simulink model "wetmodel"  (R2020b)
settings: Solver=ode45  StartTime=0.0  StopTime=inf  RelTol=1e-3  EnableMultiTasking=on
values from neighbouring files (symbols this model uses):
  controller = evalin('base','controller')    [setting_editor.m]
  s = evalin('base','s')    [GUI_MT44001.m]
undefined symbols (not defined in the file or in its folder): TS_boat
libraries: dsparch4 x6, slctrlblks x3, simulink x2, robotlib x1, dspsigops x1, aerolibutil x1
settings Model: Tag=MP_system  EnablePacing=on  Creator=Andries  LastModifiedBy=jurre
settings DataIOCC: LimitDataPoints=on  SaveFormat=Array  SignalLoggingSaveFormat=ModelDataLogs  ReturnWorkspaceOutputs=off
settings OptimizationCC: ExpressionDepthLimit=2147483647  LifeSpan=inf
settings DebuggingCC: UnderspecifiedInitializationDetection=Classic  MergeDetectMultiDrivingBlocksExec=none  SolverPrmCheckMsg=warning  FcnCallInpInsideContextMsg=warning  StateNameClashWarn=warning  SFUnexpectedBacktrackingDiag=warning  SFNoUnconditionalDefaultTransitionDiag=warning  SFExecutionAtInitializationDiag=none  ArithmeticOperatorsInVariantConditions=warning
settings HardwareCC: ProdBitPerPointer=32  ProdBitPerSizeT=32  ProdBitPerPtrDiffT=32  ProdLargestAtomicFloat=None  ProdIntDivRoundTo=Undefined  ProdEndianess=Unspecified  ProdWordSize=32  ProdHWDeviceType=32-bit Generic
settings ModelReferenceCC: PropagateSignalLabelsOutOfModel=off
settings SFSimCC: SimUseLocalCustomCode=off  CustomCodeUndefinedFunction=UseInterfaceOnly
settings RTWCC: RTWUseLocalCustomCode=off
settings CodeAppCC: StateflowObjectComments=on
settings GRTTargetCC: TargetLangStandard=C89/C90 (ANSI)  CombineOutputUpdateFcns=off  GRTInterface=on
settings ConfigComp: CovMetricSettings=dw  CovSaveCumulativeToWorkspaceVar=on  CovSaveSingleToWorkspaceVar=on  CovExternalEMLEnable=off
settings SimscapeCC: SimscapeNormalizeSystem=off

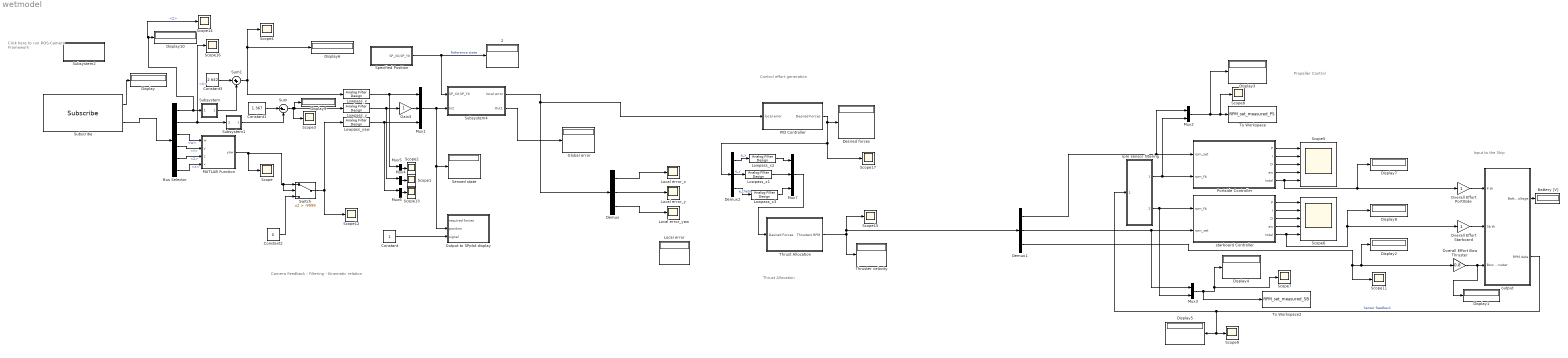
== system wetmodel ==
  note: Camera Feedback - Filtering - Kinematic relation
  note: Control effort generation
  note: Thrust Allocation
  note: Input to the Ship
  note: Propeller Control
  note: Click here to run
      | ROS-Camera Framework
  "  2" : Display
  Battery [V] : Display
  Bus Selector : BusSelector  OutputSignals=Pose.Position.Z,Pose.Position.X,Pose.Orientation.W,Pose.Orientation.Y,Pose.Orientation.Z,Pose.Orientation.X
  Constant : Constant
  Constant1 : Constant  Value=1.367
  Constant2 : Constant  Value=0
  Constant3 : Constant  Value=2.642
  Demux : Demux  Outputs=3
  Demux1 : Demux  Outputs=3
  Demux2 : Demux  Outputs=3
  Desired forces : Display
  Display{,1..10} (11 alike) : Display
  Gain3 : Gain
  Global error : Display
  Local error : Display
  "Local error_x " : Scope
  "Local error_y " : Scope
  "Local error_yaw " : Scope
  Lowpass_x{,1..3} (4 alike) : dsparch4/Analog Filter Design  method=Butterworth  filttype=Lowpass  N=1  Wlo=30  Whi=80  Rp=2  Rs=40
  Lowpass_y : dsparch4/Analog Filter Design  method=Butterworth  filttype=Lowpass  N=1  Wlo=30  Whi=80  Rp=2  Rs=40
  Lowpass_yaw : dsparch4/Analog Filter Design  method=Butterworth  filttype=Lowpass  N=8  Wlo=30  Whi=80  Rp=2  Rs=40
  MATLAB Function : MATLAB Function  TreatAsAtomicUnit=on
  Mux1 : Mux  Inputs=3
  Mux{2..6} (5 alike) : Mux  Inputs=2
  Mux7 : Mux  Inputs=3
  Output to SPplot display : Subsystem
      mask Display:
      | image(imread('spplot.JPG'))
      | port_label('input', 1, 'Req. Forces')
      | port_label('input', 2, 'Pos Update')
      | port_label('input', 3, 'signal')
  Overall Effort Bow Thruster : Gain  Gain=0.8
  Overall Effort PortISide : Gain
  Overall Effort Starboard : Gain
  PID Controller : Subsystem
  Portside Controller : Subsystem  mask{P=controller.PP, I=controller.PI, D=controller.PD, P_aw=controller.PPaw}
      mask help: Controller setting for Starboard engine
  Scope{,1..4,7..9,11..17} (15 alike) : Scope
  Scope5 : Scope  NumInputPorts=5
  Scope6 : Scope  NumInputPorts=5
  Sensed state : Display
  Specified Position : Subsystem
  Subscribe : robotlib/Subscribe  topicSource=Select from ROS network  topic=/OptiRAS/RAS_TN_RE/pose  messageType=geometry_msgs/PoseStamped  SampleTime=-1  legacyBusStruct=off  messageQueueLength=1
  Subsystem : Subsystem
  Subsystem1 : Subsystem
  Subsystem2 : Subsystem  InitFcn=|  StopFcn=set_param(gcb,'BackgroundColor','red');
      | %if ros_init==1
      | if ros.internal.Global.isNodeActive == 1
      | set_param(gcb,'BackgroundColor','green');
      | else
      | set_param(gcb,'BackgroundColor','red');
      | end
      settings: ModelCloseFcn=set_param(gcb,'BackgroundColor','red');  CloseFcn=set_param(gcb,'BackgroundColor','red');
  Subsystem4 : Subsystem
  Sum : Sum  Inputs=|+-
  Sum1 : Sum  Inputs=|++
  Switch : Switch  Criteria=u2 > Threshold  Threshold=-9999
  Thrust Allocation : Subsystem
  Thruster velocity : Display
  To Workspace : ToWorkspace  VariableName=RPM_set_measured_PS  SampleTime=-1
  To Workspace2 : ToWorkspace  VariableName=RPM_set_measured_SB  SampleTime=-1
  output : Subsystem
  rpm sensor filtering : Subsystem  mask{n_p=controller.Prpm, n_sb=controller.STrpm}
      mask prompts: n_p "Amount of holes in portside RPM sensor disc"; n_sb "Amount of holes in portside RPM sensor disc"
      mask Display:
      | port_label('output', 1, 'Ps RPM')
      | port_label('output', 2, 'SBs RPM')
  starboard Controller : Subsystem  mask{P=controller.STP, I=controller.STI, D=controller.STD, P_aw=controller.STPaw}
      mask help: Controller setting for Starboard engine
  wires:
  Specified Position/1(SP_X0,SP_Y0) -> Subsystem4/1(SP_X0,SP_Y0), "  2"/1  "Reference state"
  Mux1/1 -> Subsystem4/2(In2), Output to SPplot display/2(position), Sensed state/1
  output/2(RPM data) -> Scope9/1, Display5/1, rpm sensor filtering/1(RPM data)  "Sensor feedback"
  Portside Controller/4(aw) -> Scope5/4
  starboard Controller/3(D) -> Scope6/3
  output/1(Battery voltage) -> Battery [V]/1
  rpm sensor filtering/1(portside rpm) -> Mux2/2, Portside Controller/2(rpm_fb)
  Portside Controller/1(" P") -> Scope5/1
  rpm sensor filtering/2(starboard side rpm) -> starboard Controller/1(rpm_fb), Mux3/2
  Mux2/1 -> To Workspace/1, Scope8/1, Display3/1
  Portside Controller/3(D) -> Scope5/3
  starboard Controller/4(aw) -> Scope6/4
  Mux3/1 -> To Workspace2/1, Display4/1, Scope7/1
  Portside Controller/2(I) -> Scope5/2
  starboard Controller/2(I) -> Scope6/2
  starboard Controller/1(" P") -> Scope6/1
  Demux1/1 -> Mux2/1, Portside Controller/1(rpm_set)
  Portside Controller/5(total) -> Scope5/5, Overall Effort PortISide/1, Display7/1
  Demux1/2 -> starboard Controller/2(rpm_set), Mux3/1
  Demux1/3 -> Overall Effort Bow Thruster/1, Display2/1, Scope11/1
  Overall Effort PortISide/1 -> output/1(P th)
  Overall Effort Starboard/1 -> output/2(Sb th)
  Lowpass_x/1 -> Mux1/1, Mux5/1
  Lowpass_y/1 -> Mux4/1, Gain3/1
  Lowpass_yaw/1 -> Mux1/3, Mux6/1
  Thrust Allocation/1(Thrusters RPM) -> Demux1/1, Scope15/1, Thruster velocity/1
  PID Controller/1(Desired Forces) -> Demux2/1, Scope17/1, Desired forces/1
  Mux6/1 -> Scope13/1
  Mux4/1 -> Scope1/1
  Mux5/1 -> Scope2/1
  starboard Controller/5(total) -> Scope6/5, Overall Effort Starboard/1, Display8/1
  Overall Effort Bow Thruster/1 -> output/3("Bow thruster "), Display1/1
  Subscribe/1 -> Display/1
  Subscribe/2 -> Bus Selector/1
  Constant/1 -> Output to SPplot display/3(signal)
  Bus Selector/3 -> MATLAB Function/1(w)  "<W>"
  Bus Selector/4 -> MATLAB Function/2(y)  "<Y>"
  Bus Selector/5 -> MATLAB Function/3(z)  "<Z>"
  Bus Selector/6 -> MATLAB Function/4(x)  "<X>"
  MATLAB Function/1(yaw) -> Switch/2, Switch/1, Scope/1
  Switch/1 -> Lowpass_yaw/1, Scope12/1
  Constant2/1 -> Switch/3
  Sum/1 -> Scope3/1, Lowpass_y/1, Display9/1
  Constant1/1 -> Sum/1
  Sum1/1 -> Scope4/1, Display6/1, Lowpass_x/1
  Constant3/1 -> Sum1/1
  Bus Selector/1 -> Scope14/1, Display10/1, Subsystem/1(In1)  "<Z>"
  Bus Selector/2 -> Subsystem1/1(In1), Scope16/1  "<X>"
  Subsystem/1(Out1) -> Sum1/2
  Subsystem1/1(Out1) -> Sum/2
  Demux2/2 -> Lowpass_x1/1  "e_y"
  Demux2/3 -> Lowpass_x3/1  "e_theta"
  Lowpass_x3/1 -> Mux7/3
  Lowpass_x1/1 -> Mux7/2
  Lowpass_x2/1 -> Mux7/1
  Demux2/1 -> Lowpass_x2/1  "e_x"
  Mux7/1 -> Thrust Allocation/1(Desired Forces)
  Gain3/1 -> Mux1/2
  Subsystem4/1(local error) -> Demux/1, PID Controller/1(local error)
  Demux/1 -> "Local error_x "/1
  Demux/2 -> "Local error_y "/1
  Demux/3 -> "Local error_yaw "/1
  Subsystem4/2(Out1) -> Global error/1

== system wetmodel/Output to SPplot display ==
  required forces : Inport
  position : Inport  Port=2
  signal : Inport  Port=3
  Constant : Constant  Value=3
  Mux : Mux  Inputs=3
  Switch : Switch  Criteria=u2 > Threshold
  pos_update : S-Function  FunctionName=pos_update  Parameters=TS_wii  SFunctionDeploymentMode=off  EnableBusSupport=off
  wires:
  Mux/1 -> pos_update/1
  position/1 -> Mux/1
  required forces/1 -> Mux/3
  Switch/1 -> Mux/2
  signal/1 -> Switch/2
  Constant/1 -> Switch/1

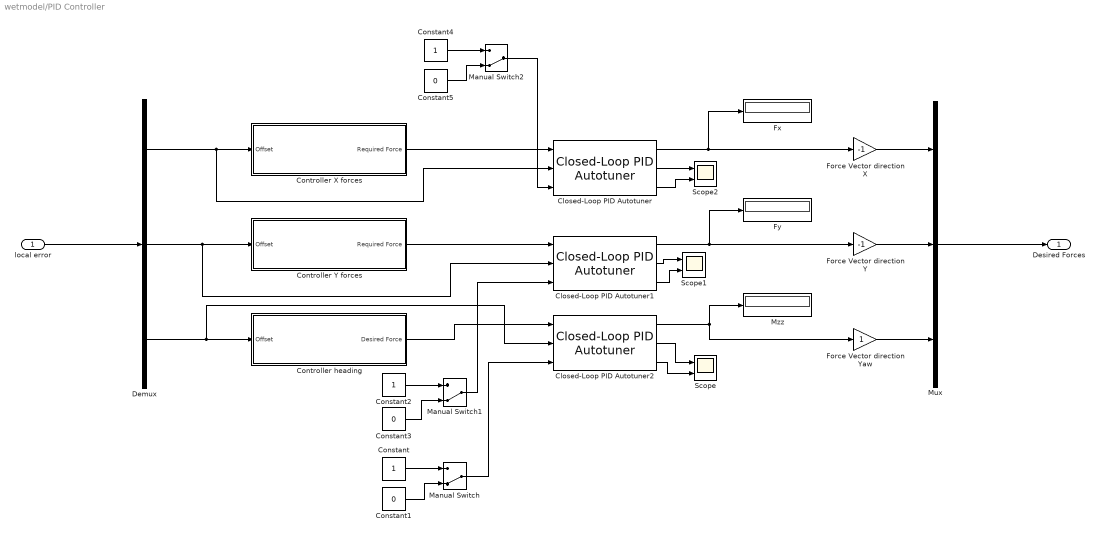
== system wetmodel/PID Controller ==
  local error : Inport
  Closed-Loop PID Autotuner : slctrlblks/Closed-Loop PID Autotuner  PIDType=PID  PIDForm=Parallel  TimeDomain=continuous-time  DiscreteTs=0.1  IntegratorFormula=Forward Euler  FilterFormula=Forward Euler  ContinuousTs=0.02  Bandwidth=1  UseExternalWC=off  TargetPM=60  UseExternalPM=off  UseExternalAchievedPM=off  PlantType=Stable  PlantSign=Positive  AmpSine=1  UseExternalAmpSine=off  UseExternalFRD=off  UseExternalU0=off  UseCompanion=off  NotDeployTuningModule=off  UsePLCCoder=off  OutputMode=control action + perturbation  BlockDataType=double  UseConnectedPID=on  blockpath=[]  tunedP=0  tunedI=0  tunedD=0  tunedN=100  tunedPM=0  EstimationWindowSize=3  UseExternalTuningParams=off  OutputChoice=VariantCandD
      settings: SourceProductBaseCode=SD
  Closed-Loop PID Autotuner1 : slctrlblks/Closed-Loop PID Autotuner  PIDType=PID  PIDForm=Parallel  TimeDomain=continuous-time  DiscreteTs=0.1  IntegratorFormula=Forward Euler  FilterFormula=Forward Euler  ContinuousTs=0.02  Bandwidth=1  UseExternalWC=off  TargetPM=60  UseExternalPM=off  UseExternalAchievedPM=off  PlantType=Stable  PlantSign=Positive  AmpSine=1  UseExternalAmpSine=off  UseExternalFRD=off  UseExternalU0=off  UseCompanion=off  NotDeployTuningModule=off  UsePLCCoder=off  OutputMode=control action + perturbation  BlockDataType=double  UseConnectedPID=on  blockpath=[]  tunedP=0  tunedI=0  tunedD=0  tunedN=100  tunedPM=0  EstimationWindowSize=3  UseExternalTuningParams=off  OutputChoice=VariantCandD
      settings: SourceProductBaseCode=SD
  Closed-Loop PID Autotuner2 : slctrlblks/Closed-Loop PID Autotuner  PIDType=PID  PIDForm=Parallel  TimeDomain=continuous-time  DiscreteTs=0.1  IntegratorFormula=Forward Euler  FilterFormula=Forward Euler  ContinuousTs=0.02  Bandwidth=1  UseExternalWC=off  TargetPM=60  UseExternalPM=off  UseExternalAchievedPM=off  PlantType=Stable  PlantSign=Positive  AmpSine=1  UseExternalAmpSine=off  UseExternalFRD=off  UseExternalU0=off  UseCompanion=off  NotDeployTuningModule=off  UsePLCCoder=off  OutputMode=control action + perturbation  BlockDataType=double  UseConnectedPID=on  blockpath=[]  tunedP=0  tunedI=0  tunedD=0  tunedN=100  tunedPM=0  EstimationWindowSize=3  UseExternalTuningParams=off  OutputChoice=VariantCandD
      settings: SourceProductBaseCode=SD
  Constant : Constant
  Constant1 : Constant  Value=0
  Constant2 : Constant
  Constant3 : Constant  Value=0
  Constant4 : Constant
  Constant5 : Constant  Value=0
  Controller X forces : Subsystem  mask{P=controller.LP, I=controller.LI, D=controller.LD, upp_lim=controller.Lmax, low_lim=controller.Lmin, P_aw=controller.LPaw}
      mask prompts: upp_lim "Upper Limit"; low_lim "Lower Limit"; P_aw "Anti wind-up gain"
  Controller Y forces : Subsystem  mask{P=controller.SP, I=controller.SI, D=controller.SD, upp_lim=controller.Smax, low_lim=controller.Smin, P_aw=controller.SPaw}
      mask prompts: upp_lim "Upper Limit"; low_lim "Lower Limit"; P_aw "Anti wind-up gain"
  Controller heading : Subsystem  mask{P=controller.HP, I=controller.HI, D=controller.HD, upp_lim=controller.Hmax, low_lim=controller.Hmin, P_aw=controller.HPaw}
      mask prompts: upp_lim "Upper Limit"; low_lim "Lower Limit"; P_aw "Anti wind-up gain"
  Demux : Demux  Outputs=3
  Force Vector direction X : Gain  Gain=-1
  Force Vector direction Y : Gain  Gain=-1
  Force Vector direction Yaw : Gain
  Fx : Display
  Fy : Display
  Manual Switch : ManualSwitch  CurrentSetting=0
  Manual Switch1 : ManualSwitch  CurrentSetting=0
  Manual Switch2 : ManualSwitch  CurrentSetting=0
  Mux : Mux  Inputs=3
  Mzz : Display
  Scope : Scope  NumInputPorts=2
  Scope1 : Scope  NumInputPorts=2
  Scope2 : Scope  NumInputPorts=2
  Desired Forces : Outport  VectorParamsAs1DForOutWhenUnconnected=off
  wires:
  Demux/3 -> Closed-Loop PID Autotuner2/2, Controller heading/1(Offset)
  Demux/2 -> Closed-Loop PID Autotuner1/2, Controller Y forces/1(Offset)
  Demux/1 -> Closed-Loop PID Autotuner/2, Controller X forces/1(Offset)
  Mux/1 -> Desired Forces/1
  local error/1 -> Demux/1
  Force Vector direction X/1 -> Mux/1
  Force Vector direction Y/1 -> Mux/2
  Force Vector direction Yaw/1 -> Mux/3
  Controller X forces/1(Required Force) -> Closed-Loop PID Autotuner/1
  Closed-Loop PID Autotuner/1 -> Fx/1, Force Vector direction X/1
  Controller Y forces/1(Required Force) -> Closed-Loop PID Autotuner1/1
  Closed-Loop PID Autotuner1/1 -> Fy/1, Force Vector direction Y/1
  Closed-Loop PID Autotuner2/1 -> Force Vector direction Yaw/1, Mzz/1
  Controller heading/1(Desired Force) -> Closed-Loop PID Autotuner2/1
  Constant/1 -> Manual Switch/1
  Constant1/1 -> Manual Switch/2
  Manual Switch/1 -> Closed-Loop PID Autotuner2/3
  Closed-Loop PID Autotuner2/2 -> Scope/1
  Closed-Loop PID Autotuner2/3 -> Scope/2
  Constant2/1 -> Manual Switch1/1
  Constant3/1 -> Manual Switch1/2
  Constant4/1 -> Manual Switch2/1
  Constant5/1 -> Manual Switch2/2
  Manual Switch2/1 -> Closed-Loop PID Autotuner/3
  Manual Switch1/1 -> Closed-Loop PID Autotuner1/3
  Closed-Loop PID Autotuner1/3 -> Scope1/2
  Closed-Loop PID Autotuner1/2 -> Scope1/1
  Closed-Loop PID Autotuner/2 -> Scope2/1
  Closed-Loop PID Autotuner/3 -> Scope2/2

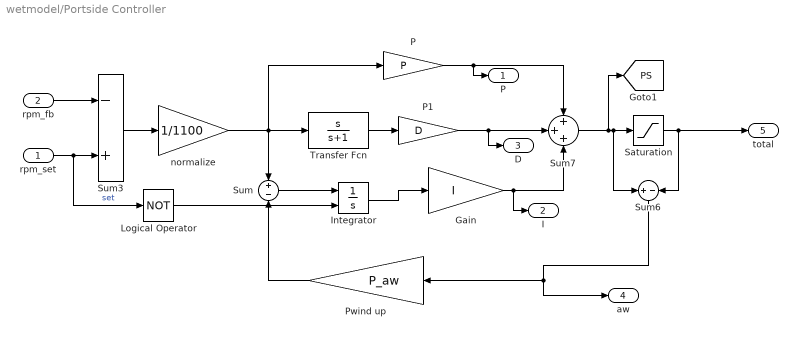
== system wetmodel/Portside Controller ==
  rpm_set : Inport
  rpm_fb : Inport  Port=2
  Gain : Gain  Gain=I  SaturateOnIntegerOverflow=on  OutDataTypeStr=Inherit: Same as input  ParamDataTypeStr=Inherit: Same as input
  Integrator : Integrator  ExternalReset=level
  Logical Operator : Logic  Operator=NOT  AllPortsSameDT=off  OutDataTypeStr=boolean
  P : Gain  Gain=P  SaturateOnIntegerOverflow=on  OutDataTypeStr=Inherit: Same as input  ParamDataTypeStr=Inherit: Same as input
  P1 : Gain  Gain=D  SaturateOnIntegerOverflow=on  OutDataTypeStr=Inherit: Same as input  ParamDataTypeStr=Inherit: Same as input
  Pwind up : Gain  Gain=P_aw  SaturateOnIntegerOverflow=on  OutDataTypeStr=Inherit: Same as input  ParamDataTypeStr=Inherit: Same as input
  Saturation : Saturate  UpperLimit=1  LowerLimit=-1
  Sum : Sum  Inputs=+|-  SaturateOnIntegerOverflow=on
  Sum3 : Sum  Inputs=-+  InputSameDT=on  SaturateOnIntegerOverflow=on  OutDataTypeStr=Inherit: Same as first input
  Sum6 : Sum  Inputs=+-  InputSameDT=on  SaturateOnIntegerOverflow=on  OutDataTypeStr=Inherit: Same as first input
  Sum7 : Sum  Inputs=+++  InputSameDT=on  SaturateOnIntegerOverflow=on  OutDataTypeStr=Inherit: Same as first input
  Transfer Fcn : TransferFcn  Numerator=[1 0]  Denominator=[1 1]
  normalize : Gain  Gain=1/1100
  " P" : Outport  VectorParamsAs1DForOutWhenUnconnected=off
  I : Outport  Port=2  VectorParamsAs1DForOutWhenUnconnected=off
  D : Outport  Port=3  VectorParamsAs1DForOutWhenUnconnected=off
  aw : Outport  Port=4  VectorParamsAs1DForOutWhenUnconnected=off
  total : Outport  Port=5  VectorParamsAs1DForOutWhenUnconnected=off
  tag scope: PS=global
  wires:
  rpm_fb/1 -> Sum3/1
  Sum/1 -> Integrator/1
  Pwind up/1 -> Sum/2
  Sum6/1 -> Pwind up/1, aw/1
  Sum7/1 -> Sum6/1, Saturation/1, [PS]
  Saturation/1 -> Sum6/2, total/1
  P/1 -> Sum7/1, " P"/1
  Sum3/1 -> normalize/1
  Integrator/1 -> Gain/1
  Gain/1 -> Sum7/3, I/1
  P1/1 -> Sum7/2, D/1
  Transfer Fcn/1 -> P1/1
  rpm_set/1 -> Sum3/2, Logical Operator/1  "set"
  normalize/1 -> Sum/1, P/1, Transfer Fcn/1
  Logical Operator/1 -> Integrator/2

== system wetmodel/Specified Position ==
  Mux : Mux  Inputs=3
  SP_X0 : Constant  Value=0
  SP_Y0 : Constant  Value=0.03
  SP_head : Constant  Value=1.3878e-16
  SP_X0,SP_Y0 : Outport  VectorParamsAs1DForOutWhenUnconnected=off
  wires:
  Mux/1 -> SP_X0,SP_Y0/1
  SP_Y0/1 -> Mux/2  "SP_Y0"
  SP_X0/1 -> Mux/1  "SP_X0"
  SP_head/1 -> Mux/3

== system wetmodel/Subsystem ==
  In1 : Inport
  Constant1 : Constant  Value=0
  Constant2 : Constant  Commented=on  Value=3.449
  Constant3 : Constant  Value=0
  Constant4 : Constant  Value=0
  Sum1 : Sum  Inputs=|++
  Switch1 : Switch  Criteria=u2 ~= 0  Threshold=-9999
  Switch2 : Switch  Criteria=u2 ~= 0  Threshold=-9999
  Out1 : Outport
  wires:
  In1/1 -> Switch2/2, Switch1/2, Switch1/1
  Constant4/1 -> Switch1/3
  Switch1/1 -> Sum1/2
  Constant1/1 -> Switch2/3
  Switch2/1 -> Sum1/1
  Sum1/1 -> Out1/1
  Constant3/1 -> Switch2/1

== system wetmodel/Subsystem1 ==
  In1 : Inport
  Constant1 : Constant  Value=0
  Constant2 : Constant  Value=0
  Constant3 : Constant  Commented=on  Value=-0.9464
  Constant4 : Constant  Value=0
  Sum1 : Sum  Inputs=|++
  Switch1 : Switch  Criteria=u2 ~= 0  Threshold=-9999
  Switch2 : Switch  Criteria=u2 ~= 0  Threshold=-9999
  Out1 : Outport
  wires:
  Constant2/1 -> Switch2/1
  Sum1/1 -> Out1/1
  Switch2/1 -> Sum1/1
  Constant1/1 -> Switch2/3
  Switch1/1 -> Sum1/2
  Constant4/1 -> Switch1/3
  In1/1 -> Switch1/1, Switch1/2, Switch2/2

== system wetmodel/Subsystem2 ==

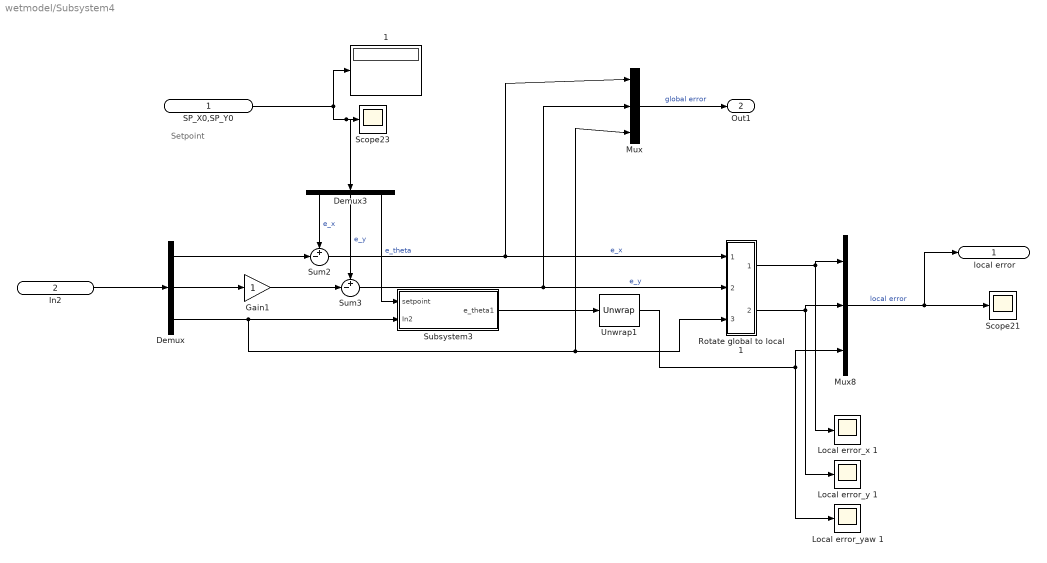
== system wetmodel/Subsystem4 ==
  note: Setpoint
  SP_X0,SP_Y0 : Inport
  In2 : Inport  Port=2
  "  1" : Display
  Demux : Demux  Outputs=3
  Demux3 : Demux  Outputs=3
  Gain1 : Gain
  Local error_x 1 : Scope
  Local error_y 1 : Scope
  Local error_yaw 1 : Scope
  Mux : Mux  Inputs=3
  Mux8 : Mux  Inputs=3
  Rotate global to local 1 : Subsystem
  Scope21 : Scope
  Scope23 : Scope
  Subsystem3 : Subsystem
  Sum2 : Sum  Inputs=+-|
  Sum3 : Sum  Inputs=+-|
  Unwrap1 : dspsigops/Unwrap  tol=pi  InputProcessing=Columns as channels (frame based)  running=off
  local error : Outport
  Out1 : Outport  Port=2
  wires:
  Demux/1 -> Sum2/2
  Unwrap1/1 -> Mux8/3, Local error_yaw 1/1
  SP_X0,SP_Y0/1 -> "  1"/1, Demux3/1, Scope23/1
  Rotate global to local 1/2(Out2) -> Mux8/2, Local error_y 1/1
  Rotate global to local 1/1(Out1) -> Mux8/1, Local error_x 1/1
  Mux8/1 -> local error/1, Scope21/1  "local error"
  Gain1/1 -> Sum3/2
  Demux3/3 -> Subsystem3/1(setpoint)  "e_theta"
  In2/1 -> Demux/1
  Demux3/2 -> Sum3/1  "e_y"
  Subsystem3/1(e_theta1) -> Unwrap1/1
  Demux/3 -> Mux/3, Rotate global to local 1/3(In3), Subsystem3/2(In2)
  Demux3/1 -> Sum2/1  "e_x"
  Demux/2 -> Gain1/1
  Sum3/1 -> Mux/2, Rotate global to local 1/2(In2)  "e_y"
  Sum2/1 -> Mux/1, Rotate global to local 1/1(In1)  "e_x"
  Mux/1 -> Out1/1  "global error"

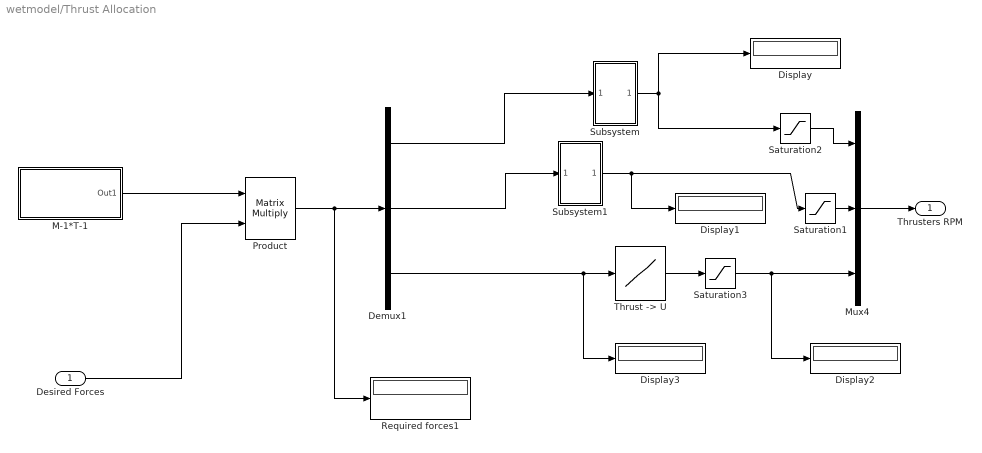
== system wetmodel/Thrust Allocation ==
  Desired Forces : Inport
  Demux1 : Demux  Outputs=3
  Display{,1..3} (4 alike) : Display
  M-1*T-1 : Subsystem
  Mux4 : Mux  Inputs=3
  Product : Product  Multiplication=Matrix(*)
  Required forces1 : Display
  Saturation1 : Saturate  UpperLimit=1100  LowerLimit=-1100
  Saturation2 : Saturate  UpperLimit=1100  LowerLimit=-1100
  Saturation3 : Saturate
  Subsystem : Subsystem
  Subsystem1 : Subsystem
  "Thrust -> U" : Lookup_n-D  NumberOfTableDimensions=1  BreakpointsForDimension1=[-1,0,0.0000001, 1]  Table=[-0.3, 0, 0.17, 0.3]  InternalRulePriority=Speed  RndMeth=Simplest  InputSameDT=on
  Thrusters RPM : Outport  VectorParamsAs1DForOutWhenUnconnected=off
  wires:
  Mux4/1 -> Thrusters RPM/1
  M-1*T-1/1(Out1) -> Product/1
  Desired Forces/1 -> Product/2
  Product/1 -> Demux1/1, Required forces1/1
  Demux1/1 -> Subsystem/1(In1)
  Saturation3/1 -> Display2/1, Mux4/3
  Demux1/2 -> Subsystem1/1(In1)
  Subsystem/1(Out1) -> Saturation2/1, Display/1
  Subsystem1/1(Out1) -> Saturation1/1, Display1/1
  Saturation2/1 -> Mux4/1
  Saturation1/1 -> Mux4/2
  Demux1/3 -> "Thrust -> U"/1, Display3/1
  "Thrust -> U"/1 -> Saturation3/1

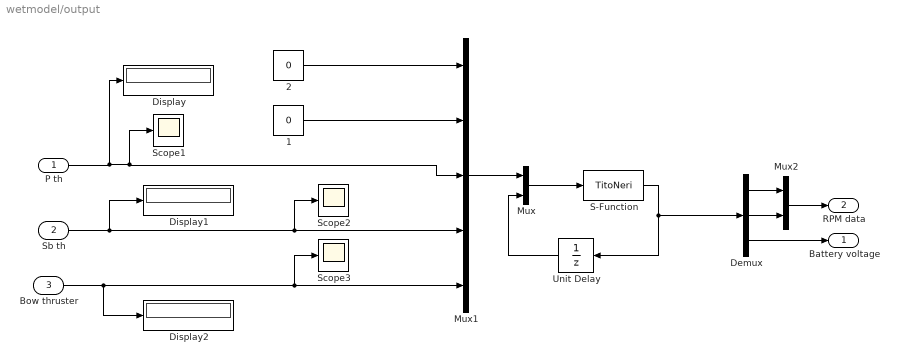
== system wetmodel/output ==
  P th : Inport
  Sb th : Inport  Port=2
  "Bow thruster " : Inport  Port=3
  1 : Constant  Value=0
  2 : Constant  Value=0
  Demux : Demux  Outputs=3
  Display : Display
  Display1 : Display
  Display2 : Display
  Mux : Mux  Inputs=2
  Mux1 : Mux  Inputs=5
  Mux2 : Mux  Inputs=2
  S-Function : S-Function  FunctionName=TitoNeri  Parameters=TS_boat,s  SFunctionDeploymentMode=off  EnableBusSupport=off
  Scope1 : Scope
  Scope2 : Scope
  Scope3 : Scope
  Unit Delay : UnitDelay  SampleTime=-1  HasFrameUpgradeWarning=on
  Battery voltage : Outport  VectorParamsAs1DForOutWhenUnconnected=off
  RPM data : Outport  Port=2  VectorParamsAs1DForOutWhenUnconnected=off
  wires:
  1/1 -> Mux1/2
  2/1 -> Mux1/1
  Mux/1 -> S-Function/1
  Unit Delay/1 -> Mux/2
  S-Function/1 -> Demux/1, Unit Delay/1
  Demux/1 -> Mux2/1
  Demux/2 -> Mux2/2
  Mux2/1 -> RPM data/1
  Demux/3 -> Battery voltage/1
  "Bow thruster "/1 -> Mux1/5, Scope3/1, Display2/1
  Sb th/1 -> Mux1/4, Scope2/1, Display1/1
  Mux1/1 -> Mux/1
  P th/1 -> Display/1, Mux1/3, Scope1/1

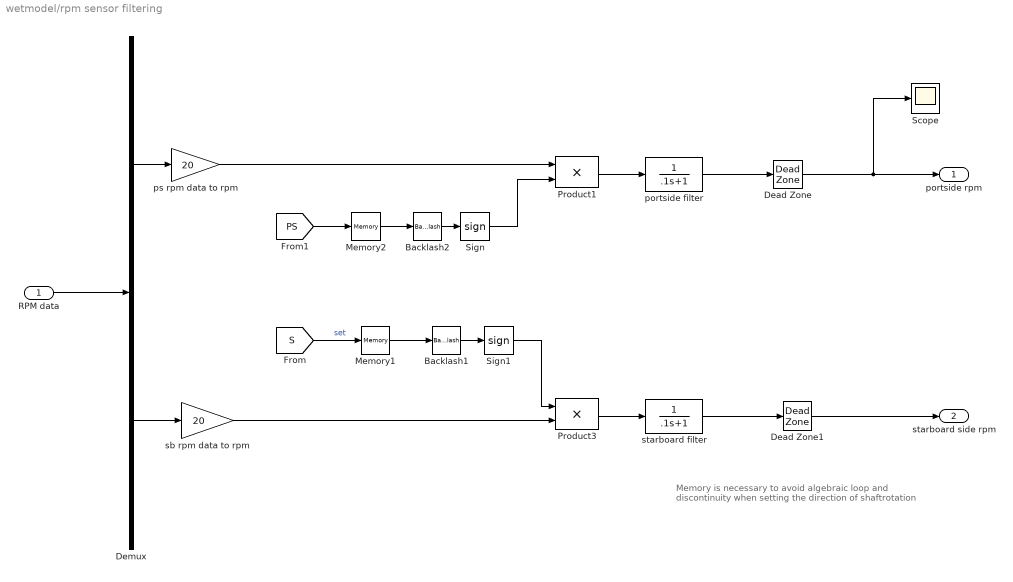
== system wetmodel/rpm sensor filtering ==
  note: Memory is necessary to avoid algebraic loop
      |  and discontinuity when setting the
      |  direction of shaftrotation
  RPM data : Inport
  " sb rpm data to rpm" : Gain  Gain=20
  Backlash1 : Backlash  BacklashWidth=.1
  Backlash2 : Backlash  BacklashWidth=.1
  Dead Zone : DeadZone  SaturateOnIntegerOverflow=on
  Dead Zone1 : DeadZone  SaturateOnIntegerOverflow=on
  Demux : Demux  Outputs=2
  Memory1 : Memory  InitialCondition=1
  Memory2 : Memory  InitialCondition=1
  Product1 : Product  InputSameDT=on  SaturateOnIntegerOverflow=on  OutDataTypeStr=Inherit: Same as first input
  Product3 : Product  InputSameDT=on  SaturateOnIntegerOverflow=on  OutDataTypeStr=Inherit: Same as first input
  Scope : Scope
  Sign : Signum
  Sign1 : Signum
  portside filter : TransferFcn  Denominator=[.1 1]
  ps rpm data to rpm : Gain  Gain=20
  starboard filter : TransferFcn  Denominator=[.1 1]
  portside rpm : Outport  VectorParamsAs1DForOutWhenUnconnected=off
  starboard side rpm : Outport  Port=2  VectorParamsAs1DForOutWhenUnconnected=off
  wires:
  RPM data/1 -> Demux/1
  Memory2/1 -> Backlash2/1
  Backlash2/1 -> Sign/1
  Product3/1 -> starboard filter/1
  Sign/1 -> Product1/2
  [PS] -> Memory2/1
  Memory1/1 -> Backlash1/1
  Backlash1/1 -> Sign1/1
  [S] -> Memory1/1  "set"
  Sign1/1 -> Product3/1
  Demux/1 -> ps rpm data to rpm/1
  Demux/2 -> " sb rpm data to rpm"/1
  Product1/1 -> portside filter/1
  " sb rpm data to rpm"/1 -> Product3/2
  starboard filter/1 -> Dead Zone1/1
  ps rpm data to rpm/1 -> Product1/1
  portside filter/1 -> Dead Zone/1
  Dead Zone/1 -> Scope/1, portside rpm/1
  Dead Zone1/1 -> starboard side rpm/1

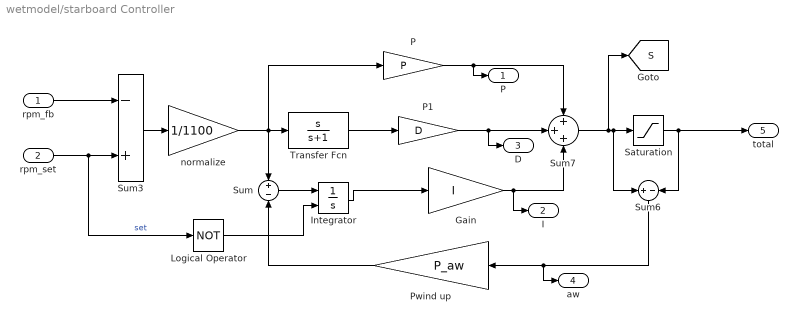
== system wetmodel/starboard Controller ==
  rpm_fb : Inport
  rpm_set : Inport  Port=2
  Gain : Gain  Gain=I  SaturateOnIntegerOverflow=on  OutDataTypeStr=Inherit: Same as input  ParamDataTypeStr=Inherit: Same as input
  Integrator : Integrator  ExternalReset=level
  Logical Operator : Logic  Operator=NOT  AllPortsSameDT=off  OutDataTypeStr=boolean
  P : Gain  Gain=P  SaturateOnIntegerOverflow=on  OutDataTypeStr=Inherit: Same as input  ParamDataTypeStr=Inherit: Same as input
  P1 : Gain  Gain=D  SaturateOnIntegerOverflow=on  OutDataTypeStr=Inherit: Same as input  ParamDataTypeStr=Inherit: Same as input
  Pwind up : Gain  Gain=P_aw  SaturateOnIntegerOverflow=on  OutDataTypeStr=Inherit: Same as input  ParamDataTypeStr=Inherit: Same as input
  Saturation : Saturate  UpperLimit=1  LowerLimit=-1
  Sum : Sum  Inputs=+|-  SaturateOnIntegerOverflow=on
  Sum3 : Sum  Inputs=-+  InputSameDT=on  SaturateOnIntegerOverflow=on  OutDataTypeStr=Inherit: Same as first input
  Sum6 : Sum  Inputs=+-  InputSameDT=on  SaturateOnIntegerOverflow=on  OutDataTypeStr=Inherit: Same as first input
  Sum7 : Sum  Inputs=+++  InputSameDT=on  SaturateOnIntegerOverflow=on  OutDataTypeStr=Inherit: Same as first input
  Transfer Fcn : TransferFcn  Numerator=[1 0]  Denominator=[1 1]
  normalize : Gain  Gain=1/1100
  " P" : Outport  VectorParamsAs1DForOutWhenUnconnected=off
  I : Outport  Port=2  VectorParamsAs1DForOutWhenUnconnected=off
  D : Outport  Port=3  VectorParamsAs1DForOutWhenUnconnected=off
  aw : Outport  Port=4  VectorParamsAs1DForOutWhenUnconnected=off
  total : Outport  Port=5  VectorParamsAs1DForOutWhenUnconnected=off
  tag scope: S=global
  wires:
  Transfer Fcn/1 -> P1/1
  P1/1 -> D/1, Sum7/2
  Gain/1 -> I/1, Sum7/3
  Integrator/1 -> Gain/1
  Sum3/1 -> normalize/1
  P/1 -> " P"/1, Sum7/1
  Saturation/1 -> Sum6/2, total/1
  Sum7/1 -> Saturation/1, Sum6/1, [S]
  Sum6/1 -> aw/1, Pwind up/1
  Pwind up/1 -> Sum/2
  Sum/1 -> Integrator/1
  rpm_fb/1 -> Sum3/1
  rpm_set/1 -> Sum3/2, Logical Operator/1  "set"
  normalize/1 -> P/1, Sum/1, Transfer Fcn/1
  Logical Operator/1 -> Integrator/2

== system wetmodel/PID Controller/Controller X forces ==
  Offset : Inport
  Add : Sum  Inputs=+++
  Derivative : TransferFcn  Numerator=[D 0]  Denominator=[0.01 1]
  Integrator : TransferFcn  Numerator=[I]  Denominator=[1 0]
  Proportional : Gain  Gain=P
  Saturation : Saturate  UpperLimit=upp_lim  LowerLimit=low_lim
  Sum : Sum  Inputs=-|+
  Sum1 : Sum  Inputs=|++
  anti wind-up gain : Gain  Gain=P_aw
  Required Force : Outport  VectorParamsAs1DForOutWhenUnconnected=off
  wires:
  anti wind-up gain/1 -> Sum1/2
  Sum/1 -> anti wind-up gain/1
  Sum1/1 -> Integrator/1
  Integrator/1 -> Add/3
  Derivative/1 -> Add/2
  Saturation/1 -> Sum/2, Required Force/1
  Add/1 -> Saturation/1, Sum/1
  Offset/1 -> Sum1/1, Derivative/1, Proportional/1
  Proportional/1 -> Add/1

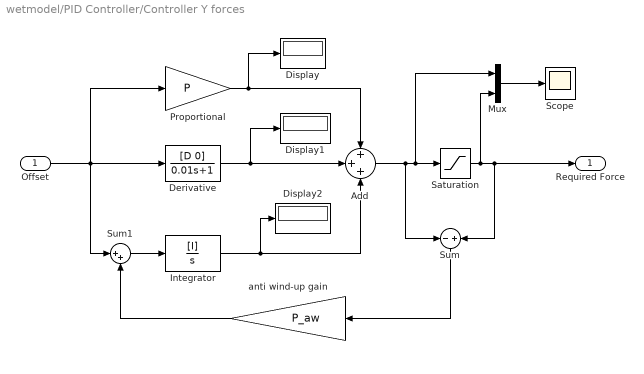
== system wetmodel/PID Controller/Controller Y forces ==
  Offset : Inport
  Add : Sum  Inputs=+++
  Derivative : TransferFcn  Numerator=[D 0]  Denominator=[0.01 1]
  Display : Display
  Display1 : Display
  Display2 : Display
  Integrator : TransferFcn  Numerator=[I]  Denominator=[1 0]
  Mux : Mux  Inputs=2
  Proportional : Gain  Gain=P
  Saturation : Saturate  UpperLimit=upp_lim  LowerLimit=low_lim
  Scope : Scope
  Sum : Sum  Inputs=-|+
  Sum1 : Sum  Inputs=|++
  anti wind-up gain : Gain  Gain=P_aw
  Required Force : Outport  VectorParamsAs1DForOutWhenUnconnected=off
  wires:
  Mux/1 -> Scope/1
  Proportional/1 -> Add/1, Display/1
  Offset/1 -> Proportional/1, Derivative/1, Sum1/1
  Add/1 -> Mux/1, Saturation/1, Sum/1
  Saturation/1 -> Required Force/1, Sum/2, Mux/2
  Derivative/1 -> Add/2, Display1/1
  Integrator/1 -> Add/3, Display2/1
  Sum1/1 -> Integrator/1
  Sum/1 -> anti wind-up gain/1
  anti wind-up gain/1 -> Sum1/2

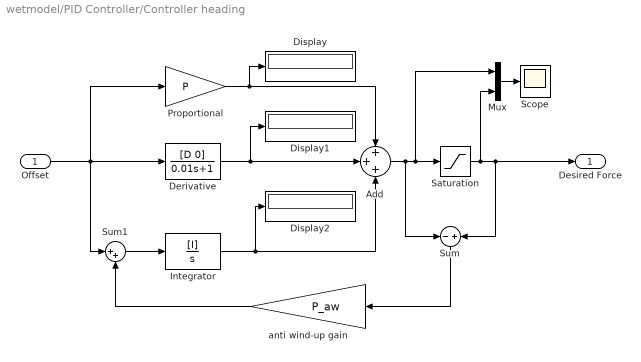
== system wetmodel/PID Controller/Controller heading ==
  Offset : Inport
  Add : Sum  Inputs=+++
  Derivative : TransferFcn  Numerator=[D 0]  Denominator=[0.01 1]
  Display : Display
  Display1 : Display
  Display2 : Display
  Integrator : TransferFcn  Numerator=[I]  Denominator=[1 0]
  Mux : Mux  Inputs=2
  Proportional : Gain  Gain=P
  Saturation : Saturate  UpperLimit=upp_lim  LowerLimit=low_lim
  Scope : Scope
  Sum : Sum  Inputs=-|+
  Sum1 : Sum  Inputs=|++
  anti wind-up gain : Gain  Gain=P_aw
  Desired Force : Outport  VectorParamsAs1DForOutWhenUnconnected=off
  wires:
  Mux/1 -> Scope/1
  Proportional/1 -> Add/1, Display/1
  Offset/1 -> Proportional/1, Derivative/1, Sum1/1
  Add/1 -> Mux/1, Saturation/1, Sum/1
  Saturation/1 -> Desired Force/1, Sum/2, Mux/2
  Derivative/1 -> Display1/1, Add/2
  Integrator/1 -> Add/3, Display2/1
  Sum1/1 -> Integrator/1
  Sum/1 -> anti wind-up gain/1
  anti wind-up gain/1 -> Sum1/2

== system wetmodel/Subsystem4/Rotate global to local 1 ==
  In1 : Inport
  In2 : Inport  Port=2
  In3 : Inport  Port=3
  Gain : Gain
  Gain4 : Gain
  Gain5 : Gain
  "Local to global x " : Subsystem
  Local to global y : Subsystem
  Out1 : Outport  VectorParamsAs1DForOutWhenUnconnected=off
  Out2 : Outport  Port=2  VectorParamsAs1DForOutWhenUnconnected=off
  wires:
  Local to global y/1(y) -> Gain5/1
  In2/1 -> Local to global y/2(Y), "Local to global x "/2(Y)
  "Local to global x "/1(x) -> Gain4/1
  In1/1 -> Local to global y/1(X), "Local to global x "/1(X)
  In3/1 -> Gain/1
  Gain/1 -> Local to global y/3(theta), "Local to global x "/3(theta)
  Gain5/1 -> Out2/1
  Gain4/1 -> Out1/1

== system wetmodel/Subsystem4/Subsystem3 ==
  setpoint : Inport
  In2 : Inport  Port=2
  Constant : Constant  Value=pi
  Gain : Gain  Gain=2
  Mod : Math  Operator=mod  SaturateOnIntegerOverflow=on
  Sum2 : Sum  Inputs=+-+
  Sum3 : Sum  Inputs=|+-
  e_theta1 : Outport
  wires:
  setpoint/1 -> Sum2/1
  Mod/1 -> Sum3/1
  Constant/1 -> Sum3/2, Gain/1, Sum2/3
  In2/1 -> Sum2/2  "theta"
  Gain/1 -> Mod/2
  Sum2/1 -> Mod/1
  Sum3/1 -> e_theta1/1  "e_theta"

== system wetmodel/Thrust Allocation/M-1*T-1 ==
  Invert 3x3 Matrix1 : aerolibutil/Invert  3x3 Matrix
  T-Matrix1 : Constant  Value=[0 1 0;1 0 1;0.47 0.08 -0.27]
  Out1 : Outport  VectorParamsAs1DForOutWhenUnconnected=off
  wires:
  T-Matrix1/1 -> Invert 3x3 Matrix1/1
  Invert 3x3 Matrix1/1 -> Out1/1

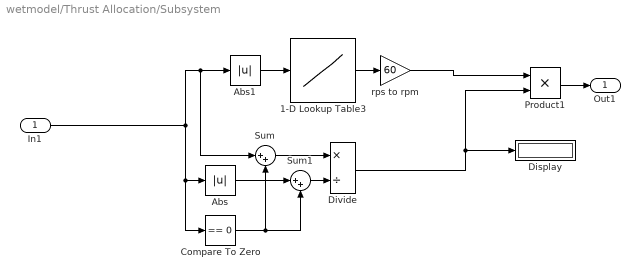
== system wetmodel/Thrust Allocation/Subsystem ==
  In1 : Inport
  1-D Lookup Table3 : Lookup_n-D  NumberOfTableDimensions=1  BreakpointsForDimension1=[0:0.01:2.5]  Table=sqrt([0:0.01:2.5]/(0.75*1000*0.06^4))+(200/60)  InternalRulePriority=Speed  RndMeth=Simplest  InputSameDT=on
  Abs : Abs
  Abs1 : Abs
  Compare To Zero : simulink/Logic and Bit Operations/Compare To Zero  relop===  OutDataTypeStr=boolean
  Display : Display
  Divide : Product  Inputs=*/
  Product1 : Product
  Sum : Sum  Inputs=|++
  Sum1 : Sum  Inputs=|++
  rps to rpm : Gain  Gain=60
  Out1 : Outport  VectorParamsAs1DForOutWhenUnconnected=off
  wires:
  rps to rpm/1 -> Product1/1
  Abs1/1 -> 1-D Lookup Table3/1
  Abs/1 -> Sum1/1
  Product1/1 -> Out1/1
  1-D Lookup Table3/1 -> rps to rpm/1
  In1/1 -> Compare To Zero/1, Abs/1, Sum/1, Abs1/1
  Divide/1 -> Display/1, Product1/2
  Sum/1 -> Divide/1
  Compare To Zero/1 -> Sum1/2, Sum/2
  Sum1/1 -> Divide/2

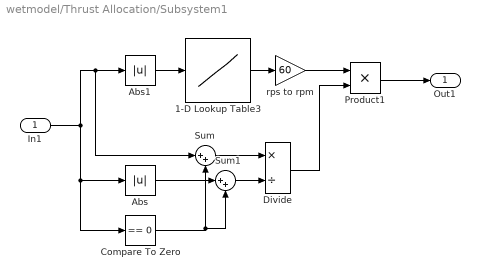
== system wetmodel/Thrust Allocation/Subsystem1 ==
  In1 : Inport
  1-D Lookup Table3 : Lookup_n-D  NumberOfTableDimensions=1  BreakpointsForDimension1=[0:0.01:2.5]  Table=sqrt([0:0.01:2.5]/(0.75*1000*0.06^4))+(200/60)  InternalRulePriority=Speed  RndMeth=Simplest  InputSameDT=on
  Abs : Abs
  Abs1 : Abs
  Compare To Zero : simulink/Logic and Bit Operations/Compare To Zero  relop===  OutDataTypeStr=boolean
  Divide : Product  Inputs=*/
  Product1 : Product
  Sum : Sum  Inputs=|++
  Sum1 : Sum  Inputs=|++
  rps to rpm : Gain  Gain=60
  Out1 : Outport  VectorParamsAs1DForOutWhenUnconnected=off
  wires:
  rps to rpm/1 -> Product1/1
  Divide/1 -> Product1/2
  Abs1/1 -> 1-D Lookup Table3/1
  Abs/1 -> Sum1/1
  Product1/1 -> Out1/1
  1-D Lookup Table3/1 -> rps to rpm/1
  In1/1 -> Compare To Zero/1, Abs/1, Sum/1, Abs1/1
  Sum/1 -> Divide/1
  Compare To Zero/1 -> Sum1/2, Sum/2
  Sum1/1 -> Divide/2

== system wetmodel/Subsystem4/Rotate global to local 1/Local to global x  ==
  X : Inport
  Y : Inport  Port=2
  theta : Inport  Port=3
  Add : Sum
  Product : Product
  Product1 : Product
  Trigonometric Function : Trigonometry  Operator=cos
  Trigonometric Function1 : Trigonometry
  x : Outport  VectorParamsAs1DForOutWhenUnconnected=off
  wires:
  Add/1 -> x/1
  Product1/1 -> Add/2
  Product/1 -> Add/1
  Y/1 -> Product1/1
  X/1 -> Product/1
  theta/1 -> Trigonometric Function1/1, Trigonometric Function/1
  Trigonometric Function1/1 -> Product1/2
  Trigonometric Function/1 -> Product/2

== system wetmodel/Subsystem4/Rotate global to local 1/Local to global y ==
  X : Inport
  Y : Inport  Port=2
  theta : Inport  Port=3
  Add : Sum  Inputs=-+
  Product : Product
  Product1 : Product
  Trigonometric Function : Trigonometry
  Trigonometric Function1 : Trigonometry  Operator=cos
  y : Outport  VectorParamsAs1DForOutWhenUnconnected=off
  wires:
  Add/1 -> y/1
  Product1/1 -> Add/2
  Product/1 -> Add/1
  Y/1 -> Product1/1
  X/1 -> Product/1
  theta/1 -> Trigonometric Function1/1, Trigonometric Function/1
  Trigonometric Function1/1 -> Product1/2
  Trigonometric Function/1 -> Product/2

== matlab function wetmodel/MATLAB Function ==
  data: w input; y input; z input; yaw output; x input
function yaw = quat2eul_VG(w,y,z,x)

%From VG MH iSCSS paper
%quatern = [ts_q4.data ts_q2.data ts_q3.data ts_q1.data]
quatern = [w,y,z,x];
%quatern = [w,x,y,z];
eulXYZ = quat2eul(quatern);
yaw = - eulXYZ(3) ;
% Change it here in case of different angle standards
